simulink model "top_level_algo"  (R2022b)
settings: Solver=FixedStepAuto  StartTime=0.0  StopTime=inf  FixedStep=1e-3  RelTol=1e-3
values from neighbouring files (symbols this model uses):
  clk_period = 8    [Cals.m]
  gear_ratio = 10    [Cals.m]
  update_rate = 0.5    [Cals.m]
  Vdd = 3    [Cals.m]
undefined symbols (not defined in the file or in its folder): sigbuilder_block
libraries: simulink x24, stm32f4xxblockslib x12, embmathops x9, arduinolib x8, dspstat3 x4, dspswit3 x2
(part 2 of 3)

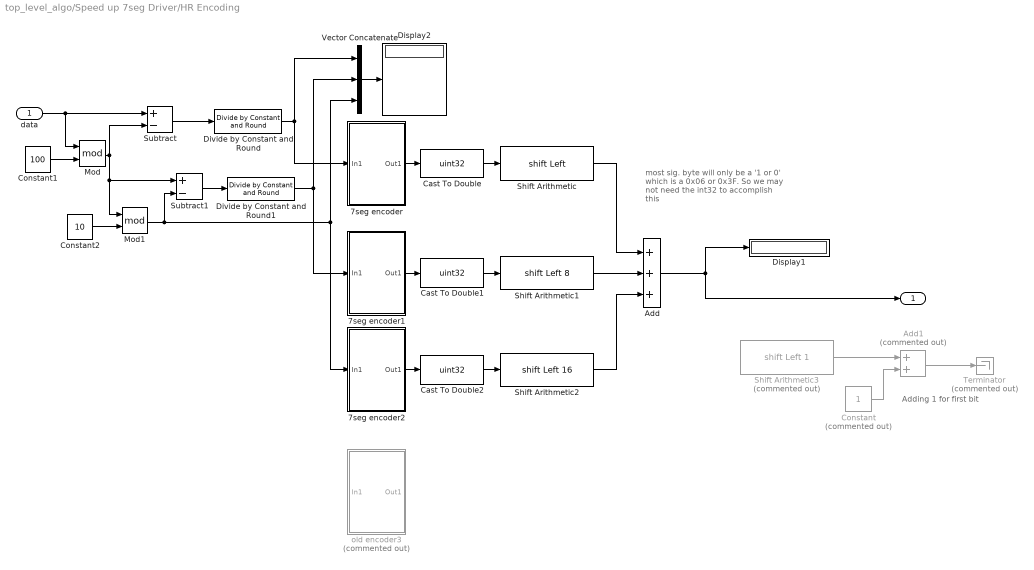
== system top_level_algo/Speed up 7seg Driver/HR Encoding ==
  note: Adding 1 for first bit
  note: most sig. byte will only be a '1 or 0' which is a 0x06 or 0x3F. So we may not need the int32 to accomplish this
  data : Inport
  7seg encoder : Subsystem
  7seg encoder1 : Subsystem
  7seg encoder2 : Subsystem
  Add : Sum  Inputs=+++
  Add1 : Sum  Commented=on
  Cast To Double : DataTypeConversion  OutDataTypeStr=uint32  SaturateOnIntegerOverflow=off  RndMeth=Floor
  Cast To Double1 : DataTypeConversion  OutDataTypeStr=uint32  SaturateOnIntegerOverflow=off  RndMeth=Floor
  Cast To Double2 : DataTypeConversion  OutDataTypeStr=uint32  SaturateOnIntegerOverflow=off  RndMeth=Floor
  Constant : Constant  Commented=on  OutDataTypeStr=uint32
  Constant1 : Constant  Value=100
  Constant2 : Constant  Value=10
  Display1 : Display
      settings: Format=hex (Stored Integer)
  Display2 : Display
  Divide by Constant and Round : embmathops/Divide by Constant and Round  Denominator=100  RoundingMethod=Floor  SimulateUsing=Code generation
  Divide by Constant and Round1 : embmathops/Divide by Constant and Round  Denominator=10  RoundingMethod=Floor  SimulateUsing=Code generation
  Mod : Math  Operator=mod
  Mod1 : Math  Operator=mod
  Shift Arithmetic : ArithShift  BitShiftDirection=Left
  Shift Arithmetic1 : ArithShift  BitShiftNumber=8  BitShiftDirection=Left
  Shift Arithmetic2 : ArithShift  BitShiftNumber=16  BitShiftDirection=Left
  Shift Arithmetic3 : ArithShift  Commented=on  BitShiftNumber=1  BitShiftDirection=Left
  Subtract : Sum  Inputs=+-
  Subtract1 : Sum  Inputs=+-
  Terminator : Terminator  Commented=on
  Vector Concatenate : Concatenate  NumInputs=3
  old encoder3 : Subsystem  Commented=on
  " " : Outport
  wires:
  Shift Arithmetic1/1 -> Add/2
  Mod1/1 -> Subtract1/2, Vector Concatenate/3, 7seg encoder2/1(In1)
  Mod/1 -> Subtract/2, Subtract1/1, Mod1/1
  7seg encoder/1(Out1) -> Cast To Double/1
  Subtract/1 -> Divide by Constant and Round/1
  Constant1/1 -> Mod/2
  Divide by Constant and Round/1 -> 7seg encoder/1(In1), Vector Concatenate/1
  Subtract1/1 -> Divide by Constant and Round1/1
  Cast To Double1/1 -> Shift Arithmetic1/1
  data/1 -> Mod/1, Subtract/1
  Add/1 -> Display1/1, " "/1
  Cast To Double/1 -> Shift Arithmetic/1
  Constant2/1 -> Mod1/2
  Vector Concatenate/1 -> Display2/1
  7seg encoder1/1(Out1) -> Cast To Double1/1
  Shift Arithmetic/1 -> Add/1
  Divide by Constant and Round1/1 -> Vector Concatenate/2, 7seg encoder1/1(In1)
  Shift Arithmetic2/1 -> Add/3
  7seg encoder2/1(Out1) -> Cast To Double2/1
  Cast To Double2/1 -> Shift Arithmetic2/1
  Constant/1 -> Add1/2
  Shift Arithmetic3/1 -> Add1/1
  Add1/1 -> Terminator/1

== system top_level_algo/Speed up 7seg Driver/clk ==
  In1 : Inport
  Cast To Single : DataTypeConversion  OutDataTypeStr=single  SaturateOnIntegerOverflow=off  RndMeth=Floor
  Compare To Constant : simulink/Logic and Bit Operations/Compare To Constant  relop=>=  const=1  OutDataTypeStr=boolean
  Constant : Constant
  Constant1 : Constant  Value=0
  Sum : Sum  Inputs=+-  InputSameDT=on  SaturateOnIntegerOverflow=on  OutDataTypeStr=Inherit: Same as first input
  Switch : Switch  Criteria=u2 > Threshold  SaturateOnIntegerOverflow=off  InputSameDT=off
  Unit Delay : UnitDelay  SampleTime=clk_period/2*1e-3  HasFrameUpgradeWarning=on
  Out1 : Outport
  wires:
  Sum/1 -> Switch/1, Out1/1
  Unit Delay/1 -> Sum/2
  In1/1 -> Cast To Single/1
  Cast To Single/1 -> Compare To Constant/1
  Constant1/1 -> Switch/3
  Compare To Constant/1 -> Switch/2
  Constant/1 -> Sum/1
  Switch/1 -> Unit Delay/1

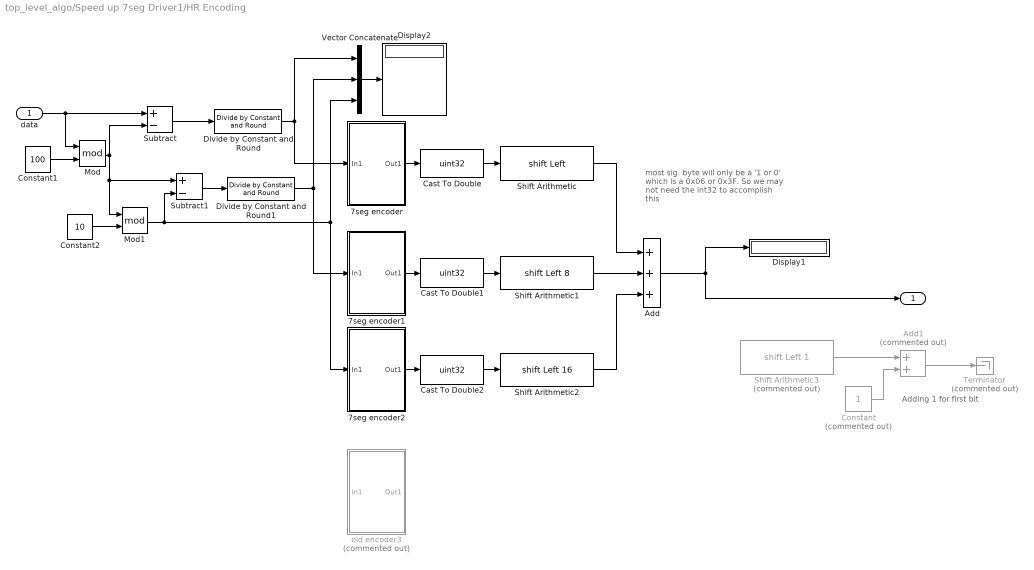
== system top_level_algo/Speed up 7seg Driver1/HR Encoding ==
  note: most sig. byte will only be a '1 or 0' which is a 0x06 or 0x3F. So we may not need the int32 to accomplish this
  note: Adding 1 for first bit
  data : Inport
  7seg encoder : Subsystem
  7seg encoder1 : Subsystem
  7seg encoder2 : Subsystem
  Add : Sum  Inputs=+++
  Add1 : Sum  Commented=on
  Cast To Double : DataTypeConversion  OutDataTypeStr=uint32  SaturateOnIntegerOverflow=off  RndMeth=Floor
  Cast To Double1 : DataTypeConversion  OutDataTypeStr=uint32  SaturateOnIntegerOverflow=off  RndMeth=Floor
  Cast To Double2 : DataTypeConversion  OutDataTypeStr=uint32  SaturateOnIntegerOverflow=off  RndMeth=Floor
  Constant : Constant  Commented=on  OutDataTypeStr=uint32
  Constant1 : Constant  Value=100
  Constant2 : Constant  Value=10
  Display1 : Display
      settings: Format=hex (Stored Integer)
  Display2 : Display
  Divide by Constant and Round : embmathops/Divide by Constant and Round  Denominator=100  RoundingMethod=Floor  SimulateUsing=Code generation
  Divide by Constant and Round1 : embmathops/Divide by Constant and Round  Denominator=10  RoundingMethod=Floor  SimulateUsing=Code generation
  Mod : Math  Operator=mod
  Mod1 : Math  Operator=mod
  Shift Arithmetic : ArithShift  BitShiftDirection=Left
  Shift Arithmetic1 : ArithShift  BitShiftNumber=8  BitShiftDirection=Left
  Shift Arithmetic2 : ArithShift  BitShiftNumber=16  BitShiftDirection=Left
  Shift Arithmetic3 : ArithShift  Commented=on  BitShiftNumber=1  BitShiftDirection=Left
  Subtract : Sum  Inputs=+-
  Subtract1 : Sum  Inputs=+-
  Terminator : Terminator  Commented=on
  Vector Concatenate : Concatenate  NumInputs=3
  old encoder3 : Subsystem  Commented=on
  " " : Outport
  wires:
  Add1/1 -> Terminator/1
  Shift Arithmetic3/1 -> Add1/1
  Constant/1 -> Add1/2
  Cast To Double2/1 -> Shift Arithmetic2/1
  7seg encoder2/1(Out1) -> Cast To Double2/1
  Shift Arithmetic2/1 -> Add/3
  Divide by Constant and Round1/1 -> 7seg encoder1/1(In1), Vector Concatenate/2
  Shift Arithmetic/1 -> Add/1
  7seg encoder1/1(Out1) -> Cast To Double1/1
  Vector Concatenate/1 -> Display2/1
  Constant2/1 -> Mod1/2
  Cast To Double/1 -> Shift Arithmetic/1
  Add/1 -> " "/1, Display1/1
  data/1 -> Subtract/1, Mod/1
  Cast To Double1/1 -> Shift Arithmetic1/1
  Subtract1/1 -> Divide by Constant and Round1/1
  Divide by Constant and Round/1 -> Vector Concatenate/1, 7seg encoder/1(In1)
  Constant1/1 -> Mod/2
  Subtract/1 -> Divide by Constant and Round/1
  7seg encoder/1(Out1) -> Cast To Double/1
  Mod/1 -> Mod1/1, Subtract1/1, Subtract/2
  Mod1/1 -> 7seg encoder2/1(In1), Vector Concatenate/3, Subtract1/2
  Shift Arithmetic1/1 -> Add/2

== system top_level_algo/Speed up 7seg Driver1/clk ==
  In1 : Inport
  Cast To Single : DataTypeConversion  OutDataTypeStr=single  SaturateOnIntegerOverflow=off  RndMeth=Floor
  Compare To Constant : simulink/Logic and Bit Operations/Compare To Constant  relop=>=  const=1  OutDataTypeStr=boolean
  Constant : Constant
  Constant1 : Constant  Value=0
  Sum : Sum  Inputs=+-  InputSameDT=on  SaturateOnIntegerOverflow=on  OutDataTypeStr=Inherit: Same as first input
  Switch : Switch  Criteria=u2 > Threshold  SaturateOnIntegerOverflow=off  InputSameDT=off
  Unit Delay : UnitDelay  SampleTime=clk_period/2*1e-3  HasFrameUpgradeWarning=on
  Out1 : Outport
  wires:
  Switch/1 -> Unit Delay/1
  Constant/1 -> Sum/1
  Compare To Constant/1 -> Switch/2
  Constant1/1 -> Switch/3
  Cast To Single/1 -> Compare To Constant/1
  In1/1 -> Cast To Single/1
  Unit Delay/1 -> Sum/2
  Sum/1 -> Out1/1, Switch/1

== system top_level_algo/7seg Driver/HR Encoding/7seg encoder ==
  In1 : Inport
  If Action Subsystem : Subsystem  TreatAsAtomicUnit=on
  If Action Subsystem1 : Subsystem  TreatAsAtomicUnit=on
  If Action Subsystem10 : Subsystem  TreatAsAtomicUnit=on
  If Action Subsystem2 : Subsystem  TreatAsAtomicUnit=on
  If Action Subsystem3 : Subsystem  TreatAsAtomicUnit=on
  If Action Subsystem4 : Subsystem  TreatAsAtomicUnit=on
  If Action Subsystem5 : Subsystem  TreatAsAtomicUnit=on
  If Action Subsystem6 : Subsystem  TreatAsAtomicUnit=on
  If Action Subsystem7 : Subsystem  TreatAsAtomicUnit=on
  If Action Subsystem8 : Subsystem  TreatAsAtomicUnit=on
  Merge : Merge  Inputs=10
  Switch Case : SwitchCase  CaseConditions={0,1,2,3,4,5,6,7,8,9}  ShowDefaultCase=off
  Out1 : Outport
  wires:
  If Action Subsystem3/1(Out1) -> Merge/4
  Switch Case/2 -> If Action Subsystem1/Action
  Switch Case/5 -> If Action Subsystem4/Action
  Switch Case/9 -> If Action Subsystem8/Action
  If Action Subsystem7/1(Out1) -> Merge/8
  Switch Case/6 -> If Action Subsystem5/Action
  If Action Subsystem4/1(Out1) -> Merge/5
  Switch Case/4 -> If Action Subsystem3/Action
  Switch Case/3 -> If Action Subsystem2/Action
  Switch Case/10 -> If Action Subsystem10/Action
  Switch Case/8 -> If Action Subsystem7/Action
  Switch Case/7 -> If Action Subsystem6/Action
  Switch Case/1 -> If Action Subsystem/Action
  If Action Subsystem6/1(Out1) -> Merge/7
  If Action Subsystem8/1(Out1) -> Merge/9
  If Action Subsystem5/1(Out1) -> Merge/6
  If Action Subsystem2/1(Out1) -> Merge/3
  If Action Subsystem10/1(Out1) -> Merge/10
  If Action Subsystem/1(Out1) -> Merge/1
  If Action Subsystem1/1(Out1) -> Merge/2
  In1/1 -> Switch Case/1
  Merge/1 -> Out1/1

== system top_level_algo/7seg Driver/HR Encoding/7seg encoder1 ==
  In1 : Inport
  If Action Subsystem : Subsystem  TreatAsAtomicUnit=on
  If Action Subsystem1 : Subsystem  TreatAsAtomicUnit=on
  If Action Subsystem10 : Subsystem  TreatAsAtomicUnit=on
  If Action Subsystem2 : Subsystem  TreatAsAtomicUnit=on
  If Action Subsystem3 : Subsystem  TreatAsAtomicUnit=on
  If Action Subsystem4 : Subsystem  TreatAsAtomicUnit=on
  If Action Subsystem5 : Subsystem  TreatAsAtomicUnit=on
  If Action Subsystem6 : Subsystem  TreatAsAtomicUnit=on
  If Action Subsystem7 : Subsystem  TreatAsAtomicUnit=on
  If Action Subsystem8 : Subsystem  TreatAsAtomicUnit=on
  Merge : Merge  Inputs=10
  Switch Case : SwitchCase  CaseConditions={0,1,2,3,4,5,6,7,8,9}  ShowDefaultCase=off
  Out1 : Outport
  wires:
  If Action Subsystem3/1(Out1) -> Merge/4
  Switch Case/2 -> If Action Subsystem1/Action
  Switch Case/5 -> If Action Subsystem4/Action
  Switch Case/9 -> If Action Subsystem8/Action
  If Action Subsystem7/1(Out1) -> Merge/8
  Switch Case/6 -> If Action Subsystem5/Action
  If Action Subsystem4/1(Out1) -> Merge/5
  Switch Case/4 -> If Action Subsystem3/Action
  Switch Case/3 -> If Action Subsystem2/Action
  Switch Case/10 -> If Action Subsystem10/Action
  Switch Case/8 -> If Action Subsystem7/Action
  Switch Case/7 -> If Action Subsystem6/Action
  Switch Case/1 -> If Action Subsystem/Action
  If Action Subsystem6/1(Out1) -> Merge/7
  If Action Subsystem8/1(Out1) -> Merge/9
  If Action Subsystem5/1(Out1) -> Merge/6
  If Action Subsystem2/1(Out1) -> Merge/3
  If Action Subsystem10/1(Out1) -> Merge/10
  If Action Subsystem/1(Out1) -> Merge/1
  If Action Subsystem1/1(Out1) -> Merge/2
  In1/1 -> Switch Case/1
  Merge/1 -> Out1/1

== system top_level_algo/7seg Driver/HR Encoding/7seg encoder2 ==
  In1 : Inport
  If Action Subsystem : Subsystem  TreatAsAtomicUnit=on
  If Action Subsystem1 : Subsystem  TreatAsAtomicUnit=on
  If Action Subsystem10 : Subsystem  TreatAsAtomicUnit=on
  If Action Subsystem2 : Subsystem  TreatAsAtomicUnit=on
  If Action Subsystem3 : Subsystem  TreatAsAtomicUnit=on
  If Action Subsystem4 : Subsystem  TreatAsAtomicUnit=on
  If Action Subsystem5 : Subsystem  TreatAsAtomicUnit=on
  If Action Subsystem6 : Subsystem  TreatAsAtomicUnit=on
  If Action Subsystem7 : Subsystem  TreatAsAtomicUnit=on
  If Action Subsystem8 : Subsystem  TreatAsAtomicUnit=on
  Merge : Merge  Inputs=10
  Switch Case : SwitchCase  CaseConditions={0,1,2,3,4,5,6,7,8,9}  ShowDefaultCase=off
  Out1 : Outport
  wires:
  If Action Subsystem3/1(Out1) -> Merge/4
  Switch Case/2 -> If Action Subsystem1/Action
  Switch Case/5 -> If Action Subsystem4/Action
  Switch Case/9 -> If Action Subsystem8/Action
  If Action Subsystem7/1(Out1) -> Merge/8
  Switch Case/6 -> If Action Subsystem5/Action
  If Action Subsystem4/1(Out1) -> Merge/5
  Switch Case/4 -> If Action Subsystem3/Action
  Switch Case/3 -> If Action Subsystem2/Action
  Switch Case/10 -> If Action Subsystem10/Action
  Switch Case/8 -> If Action Subsystem7/Action
  Switch Case/7 -> If Action Subsystem6/Action
  Switch Case/1 -> If Action Subsystem/Action
  If Action Subsystem6/1(Out1) -> Merge/7
  If Action Subsystem8/1(Out1) -> Merge/9
  If Action Subsystem5/1(Out1) -> Merge/6
  If Action Subsystem2/1(Out1) -> Merge/3
  If Action Subsystem10/1(Out1) -> Merge/10
  If Action Subsystem/1(Out1) -> Merge/1
  If Action Subsystem1/1(Out1) -> Merge/2
  In1/1 -> Switch Case/1
  Merge/1 -> Out1/1

== system top_level_algo/7seg Driver/HR Encoding/old encoder3 ==
  In1 : Inport
  If Action Subsystem : Subsystem  TreatAsAtomicUnit=on
  If Action Subsystem1 : Subsystem  TreatAsAtomicUnit=on
  If Action Subsystem10 : Subsystem  TreatAsAtomicUnit=on
  If Action Subsystem2 : Subsystem  TreatAsAtomicUnit=on
  If Action Subsystem3 : Subsystem  TreatAsAtomicUnit=on
  If Action Subsystem4 : Subsystem  TreatAsAtomicUnit=on
  If Action Subsystem5 : Subsystem  TreatAsAtomicUnit=on
  If Action Subsystem6 : Subsystem  TreatAsAtomicUnit=on
  If Action Subsystem7 : Subsystem  TreatAsAtomicUnit=on
  If Action Subsystem8 : Subsystem  TreatAsAtomicUnit=on
  Merge : Merge  Inputs=10
  Switch Case : SwitchCase  CaseConditions={0,1,2,3,4,5,6,7,8,9}  ShowDefaultCase=off
  Out1 : Outport
  wires:
  If Action Subsystem3/1(Out1) -> Merge/4
  Switch Case/2 -> If Action Subsystem1/Action
  Switch Case/5 -> If Action Subsystem4/Action
  Switch Case/9 -> If Action Subsystem8/Action
  If Action Subsystem7/1(Out1) -> Merge/8
  Switch Case/6 -> If Action Subsystem5/Action
  If Action Subsystem4/1(Out1) -> Merge/5
  Switch Case/4 -> If Action Subsystem3/Action
  Switch Case/3 -> If Action Subsystem2/Action
  Switch Case/10 -> If Action Subsystem10/Action
  Switch Case/8 -> If Action Subsystem7/Action
  Switch Case/7 -> If Action Subsystem6/Action
  Switch Case/1 -> If Action Subsystem/Action
  If Action Subsystem6/1(Out1) -> Merge/7
  If Action Subsystem8/1(Out1) -> Merge/9
  If Action Subsystem5/1(Out1) -> Merge/6
  If Action Subsystem2/1(Out1) -> Merge/3
  If Action Subsystem10/1(Out1) -> Merge/10
  If Action Subsystem/1(Out1) -> Merge/1
  If Action Subsystem1/1(Out1) -> Merge/2
  In1/1 -> Switch Case/1
  Merge/1 -> Out1/1

== system top_level_algo/7seg Driver2/HR Encoding/7seg encoder ==
  In1 : Inport
  If Action Subsystem : Subsystem  TreatAsAtomicUnit=on
  If Action Subsystem1 : Subsystem  TreatAsAtomicUnit=on
  If Action Subsystem10 : Subsystem  TreatAsAtomicUnit=on
  If Action Subsystem2 : Subsystem  TreatAsAtomicUnit=on
  If Action Subsystem3 : Subsystem  TreatAsAtomicUnit=on
  If Action Subsystem4 : Subsystem  TreatAsAtomicUnit=on
  If Action Subsystem5 : Subsystem  TreatAsAtomicUnit=on
  If Action Subsystem6 : Subsystem  TreatAsAtomicUnit=on
  If Action Subsystem7 : Subsystem  TreatAsAtomicUnit=on
  If Action Subsystem8 : Subsystem  TreatAsAtomicUnit=on
  Merge : Merge  Inputs=10
  Switch Case : SwitchCase  CaseConditions={0,1,2,3,4,5,6,7,8,9}  ShowDefaultCase=off
  Out1 : Outport
  wires:
  If Action Subsystem3/1(Out1) -> Merge/4
  Switch Case/2 -> If Action Subsystem1/Action
  Switch Case/5 -> If Action Subsystem4/Action
  Switch Case/9 -> If Action Subsystem8/Action
  If Action Subsystem7/1(Out1) -> Merge/8
  Switch Case/6 -> If Action Subsystem5/Action
  If Action Subsystem4/1(Out1) -> Merge/5
  Switch Case/4 -> If Action Subsystem3/Action
  Switch Case/3 -> If Action Subsystem2/Action
  Switch Case/10 -> If Action Subsystem10/Action
  Switch Case/8 -> If Action Subsystem7/Action
  Switch Case/7 -> If Action Subsystem6/Action
  Switch Case/1 -> If Action Subsystem/Action
  If Action Subsystem6/1(Out1) -> Merge/7
  If Action Subsystem8/1(Out1) -> Merge/9
  If Action Subsystem5/1(Out1) -> Merge/6
  If Action Subsystem2/1(Out1) -> Merge/3
  If Action Subsystem10/1(Out1) -> Merge/10
  If Action Subsystem/1(Out1) -> Merge/1
  If Action Subsystem1/1(Out1) -> Merge/2
  In1/1 -> Switch Case/1
  Merge/1 -> Out1/1

== system top_level_algo/7seg Driver2/HR Encoding/7seg encoder1 ==
  In1 : Inport
  If Action Subsystem : Subsystem  TreatAsAtomicUnit=on
  If Action Subsystem1 : Subsystem  TreatAsAtomicUnit=on
  If Action Subsystem10 : Subsystem  TreatAsAtomicUnit=on
  If Action Subsystem2 : Subsystem  TreatAsAtomicUnit=on
  If Action Subsystem3 : Subsystem  TreatAsAtomicUnit=on
  If Action Subsystem4 : Subsystem  TreatAsAtomicUnit=on
  If Action Subsystem5 : Subsystem  TreatAsAtomicUnit=on
  If Action Subsystem6 : Subsystem  TreatAsAtomicUnit=on
  If Action Subsystem7 : Subsystem  TreatAsAtomicUnit=on
  If Action Subsystem8 : Subsystem  TreatAsAtomicUnit=on
  Merge : Merge  Inputs=10
  Switch Case : SwitchCase  CaseConditions={0,1,2,3,4,5,6,7,8,9}  ShowDefaultCase=off
  Out1 : Outport
  wires:
  If Action Subsystem3/1(Out1) -> Merge/4
  Switch Case/2 -> If Action Subsystem1/Action
  Switch Case/5 -> If Action Subsystem4/Action
  Switch Case/9 -> If Action Subsystem8/Action
  If Action Subsystem7/1(Out1) -> Merge/8
  Switch Case/6 -> If Action Subsystem5/Action
  If Action Subsystem4/1(Out1) -> Merge/5
  Switch Case/4 -> If Action Subsystem3/Action
  Switch Case/3 -> If Action Subsystem2/Action
  Switch Case/10 -> If Action Subsystem10/Action
  Switch Case/8 -> If Action Subsystem7/Action
  Switch Case/7 -> If Action Subsystem6/Action
  Switch Case/1 -> If Action Subsystem/Action
  If Action Subsystem6/1(Out1) -> Merge/7
  If Action Subsystem8/1(Out1) -> Merge/9
  If Action Subsystem5/1(Out1) -> Merge/6
  If Action Subsystem2/1(Out1) -> Merge/3
  If Action Subsystem10/1(Out1) -> Merge/10
  If Action Subsystem/1(Out1) -> Merge/1
  If Action Subsystem1/1(Out1) -> Merge/2
  In1/1 -> Switch Case/1
  Merge/1 -> Out1/1

== system top_level_algo/7seg Driver2/HR Encoding/7seg encoder2 ==
  In1 : Inport
  If Action Subsystem : Subsystem  TreatAsAtomicUnit=on
  If Action Subsystem1 : Subsystem  TreatAsAtomicUnit=on
  If Action Subsystem10 : Subsystem  TreatAsAtomicUnit=on
  If Action Subsystem2 : Subsystem  TreatAsAtomicUnit=on
  If Action Subsystem3 : Subsystem  TreatAsAtomicUnit=on
  If Action Subsystem4 : Subsystem  TreatAsAtomicUnit=on
  If Action Subsystem5 : Subsystem  TreatAsAtomicUnit=on
  If Action Subsystem6 : Subsystem  TreatAsAtomicUnit=on
  If Action Subsystem7 : Subsystem  TreatAsAtomicUnit=on
  If Action Subsystem8 : Subsystem  TreatAsAtomicUnit=on
  Merge : Merge  Inputs=10
  Switch Case : SwitchCase  CaseConditions={0,1,2,3,4,5,6,7,8,9}  ShowDefaultCase=off
  Out1 : Outport
  wires:
  If Action Subsystem3/1(Out1) -> Merge/4
  Switch Case/2 -> If Action Subsystem1/Action
  Switch Case/5 -> If Action Subsystem4/Action
  Switch Case/9 -> If Action Subsystem8/Action
  If Action Subsystem7/1(Out1) -> Merge/8
  Switch Case/6 -> If Action Subsystem5/Action
  If Action Subsystem4/1(Out1) -> Merge/5
  Switch Case/4 -> If Action Subsystem3/Action
  Switch Case/3 -> If Action Subsystem2/Action
  Switch Case/10 -> If Action Subsystem10/Action
  Switch Case/8 -> If Action Subsystem7/Action
  Switch Case/7 -> If Action Subsystem6/Action
  Switch Case/1 -> If Action Subsystem/Action
  If Action Subsystem6/1(Out1) -> Merge/7
  If Action Subsystem8/1(Out1) -> Merge/9
  If Action Subsystem5/1(Out1) -> Merge/6
  If Action Subsystem2/1(Out1) -> Merge/3
  If Action Subsystem10/1(Out1) -> Merge/10
  If Action Subsystem/1(Out1) -> Merge/1
  If Action Subsystem1/1(Out1) -> Merge/2
  In1/1 -> Switch Case/1
  Merge/1 -> Out1/1

== system top_level_algo/7seg Driver2/HR Encoding/old encoder3 ==
  In1 : Inport
  If Action Subsystem : Subsystem  TreatAsAtomicUnit=on
  If Action Subsystem1 : Subsystem  TreatAsAtomicUnit=on
  If Action Subsystem10 : Subsystem  TreatAsAtomicUnit=on
  If Action Subsystem2 : Subsystem  TreatAsAtomicUnit=on
  If Action Subsystem3 : Subsystem  TreatAsAtomicUnit=on
  If Action Subsystem4 : Subsystem  TreatAsAtomicUnit=on
  If Action Subsystem5 : Subsystem  TreatAsAtomicUnit=on
  If Action Subsystem6 : Subsystem  TreatAsAtomicUnit=on
  If Action Subsystem7 : Subsystem  TreatAsAtomicUnit=on
  If Action Subsystem8 : Subsystem  TreatAsAtomicUnit=on
  Merge : Merge  Inputs=10
  Switch Case : SwitchCase  CaseConditions={0,1,2,3,4,5,6,7,8,9}  ShowDefaultCase=off
  Out1 : Outport
  wires:
  If Action Subsystem3/1(Out1) -> Merge/4
  Switch Case/2 -> If Action Subsystem1/Action
  Switch Case/5 -> If Action Subsystem4/Action
  Switch Case/9 -> If Action Subsystem8/Action
  If Action Subsystem7/1(Out1) -> Merge/8
  Switch Case/6 -> If Action Subsystem5/Action
  If Action Subsystem4/1(Out1) -> Merge/5
  Switch Case/4 -> If Action Subsystem3/Action
  Switch Case/3 -> If Action Subsystem2/Action
  Switch Case/10 -> If Action Subsystem10/Action
  Switch Case/8 -> If Action Subsystem7/Action
  Switch Case/7 -> If Action Subsystem6/Action
  Switch Case/1 -> If Action Subsystem/Action
  If Action Subsystem6/1(Out1) -> Merge/7
  If Action Subsystem8/1(Out1) -> Merge/9
  If Action Subsystem5/1(Out1) -> Merge/6
  If Action Subsystem2/1(Out1) -> Merge/3
  If Action Subsystem10/1(Out1) -> Merge/10
  If Action Subsystem/1(Out1) -> Merge/1
  If Action Subsystem1/1(Out1) -> Merge/2
  In1/1 -> Switch Case/1
  Merge/1 -> Out1/1

== system top_level_algo/Hardware Hiding/force min to zero/If Action Subsystem ==
  In1 : Inport
  Action Port : ActionPort  ActionPortLabel=if(u1 < 0)
  Out1 : Outport
  wires:
  In1/1 -> Out1/1

== system top_level_algo/Hardware Hiding/force min to zero/If Action Subsystem1 ==
  In1 : Inport
  Action Port : ActionPort  ActionPortLabel=else
  Out1 : Outport
  wires:
  In1/1 -> Out1/1

== system top_level_algo/MinMax/force min to zero/If Action Subsystem ==
  In1 : Inport
  Action Port : ActionPort  ActionPortLabel=if(u1 < 0)
  Out1 : Outport
  wires:
  In1/1 -> Out1/1

== system top_level_algo/MinMax/force min to zero/If Action Subsystem1 ==
  In1 : Inport
  Action Port : ActionPort  ActionPortLabel=else
  Out1 : Outport
  wires:
  In1/1 -> Out1/1

== system top_level_algo/Speed up 7seg Driver/HR Encoding/7seg encoder ==
  In1 : Inport
  If Action Subsystem : Subsystem  TreatAsAtomicUnit=on
  If Action Subsystem1 : Subsystem  TreatAsAtomicUnit=on
  If Action Subsystem10 : Subsystem  TreatAsAtomicUnit=on
  If Action Subsystem2 : Subsystem  TreatAsAtomicUnit=on
  If Action Subsystem3 : Subsystem  TreatAsAtomicUnit=on
  If Action Subsystem4 : Subsystem  TreatAsAtomicUnit=on
  If Action Subsystem5 : Subsystem  TreatAsAtomicUnit=on
  If Action Subsystem6 : Subsystem  TreatAsAtomicUnit=on
  If Action Subsystem7 : Subsystem  TreatAsAtomicUnit=on
  If Action Subsystem8 : Subsystem  TreatAsAtomicUnit=on
  Merge : Merge  Inputs=10
  Switch Case : SwitchCase  CaseConditions={0,1,2,3,4,5,6,7,8,9}  ShowDefaultCase=off
  Out1 : Outport
  wires:
  If Action Subsystem3/1(Out1) -> Merge/4
  Switch Case/2 -> If Action Subsystem1/Action
  Switch Case/5 -> If Action Subsystem4/Action
  Switch Case/9 -> If Action Subsystem8/Action
  If Action Subsystem7/1(Out1) -> Merge/8
  Switch Case/6 -> If Action Subsystem5/Action
  If Action Subsystem4/1(Out1) -> Merge/5
  Switch Case/4 -> If Action Subsystem3/Action
  Switch Case/3 -> If Action Subsystem2/Action
  Switch Case/10 -> If Action Subsystem10/Action
  Switch Case/8 -> If Action Subsystem7/Action
  Switch Case/7 -> If Action Subsystem6/Action
  Switch Case/1 -> If Action Subsystem/Action
  If Action Subsystem6/1(Out1) -> Merge/7
  If Action Subsystem8/1(Out1) -> Merge/9
  If Action Subsystem5/1(Out1) -> Merge/6
  If Action Subsystem2/1(Out1) -> Merge/3
  If Action Subsystem10/1(Out1) -> Merge/10
  If Action Subsystem/1(Out1) -> Merge/1
  If Action Subsystem1/1(Out1) -> Merge/2
  In1/1 -> Switch Case/1
  Merge/1 -> Out1/1

== system top_level_algo/Speed up 7seg Driver/HR Encoding/7seg encoder1 ==
  In1 : Inport
  If Action Subsystem : Subsystem  TreatAsAtomicUnit=on
  If Action Subsystem1 : Subsystem  TreatAsAtomicUnit=on
  If Action Subsystem10 : Subsystem  TreatAsAtomicUnit=on
  If Action Subsystem2 : Subsystem  TreatAsAtomicUnit=on
  If Action Subsystem3 : Subsystem  TreatAsAtomicUnit=on
  If Action Subsystem4 : Subsystem  TreatAsAtomicUnit=on
  If Action Subsystem5 : Subsystem  TreatAsAtomicUnit=on
  If Action Subsystem6 : Subsystem  TreatAsAtomicUnit=on
  If Action Subsystem7 : Subsystem  TreatAsAtomicUnit=on
  If Action Subsystem8 : Subsystem  TreatAsAtomicUnit=on
  Merge : Merge  Inputs=10
  Switch Case : SwitchCase  CaseConditions={0,1,2,3,4,5,6,7,8,9}  ShowDefaultCase=off
  Out1 : Outport
  wires:
  If Action Subsystem3/1(Out1) -> Merge/4
  Switch Case/2 -> If Action Subsystem1/Action
  Switch Case/5 -> If Action Subsystem4/Action
  Switch Case/9 -> If Action Subsystem8/Action
  If Action Subsystem7/1(Out1) -> Merge/8
  Switch Case/6 -> If Action Subsystem5/Action
  If Action Subsystem4/1(Out1) -> Merge/5
  Switch Case/4 -> If Action Subsystem3/Action
  Switch Case/3 -> If Action Subsystem2/Action
  Switch Case/10 -> If Action Subsystem10/Action
  Switch Case/8 -> If Action Subsystem7/Action
  Switch Case/7 -> If Action Subsystem6/Action
  Switch Case/1 -> If Action Subsystem/Action
  If Action Subsystem6/1(Out1) -> Merge/7
  If Action Subsystem8/1(Out1) -> Merge/9
  If Action Subsystem5/1(Out1) -> Merge/6
  If Action Subsystem2/1(Out1) -> Merge/3
  If Action Subsystem10/1(Out1) -> Merge/10
  If Action Subsystem/1(Out1) -> Merge/1
  If Action Subsystem1/1(Out1) -> Merge/2
  In1/1 -> Switch Case/1
  Merge/1 -> Out1/1

== system top_level_algo/Speed up 7seg Driver/HR Encoding/7seg encoder2 ==
  In1 : Inport
  If Action Subsystem : Subsystem  TreatAsAtomicUnit=on
  If Action Subsystem1 : Subsystem  TreatAsAtomicUnit=on
  If Action Subsystem10 : Subsystem  TreatAsAtomicUnit=on
  If Action Subsystem2 : Subsystem  TreatAsAtomicUnit=on
  If Action Subsystem3 : Subsystem  TreatAsAtomicUnit=on
  If Action Subsystem4 : Subsystem  TreatAsAtomicUnit=on
  If Action Subsystem5 : Subsystem  TreatAsAtomicUnit=on
  If Action Subsystem6 : Subsystem  TreatAsAtomicUnit=on
  If Action Subsystem7 : Subsystem  TreatAsAtomicUnit=on
  If Action Subsystem8 : Subsystem  TreatAsAtomicUnit=on
  Merge : Merge  Inputs=10
  Switch Case : SwitchCase  CaseConditions={0,1,2,3,4,5,6,7,8,9}  ShowDefaultCase=off
  Out1 : Outport
  wires:
  If Action Subsystem3/1(Out1) -> Merge/4
  Switch Case/2 -> If Action Subsystem1/Action
  Switch Case/5 -> If Action Subsystem4/Action
  Switch Case/9 -> If Action Subsystem8/Action
  If Action Subsystem7/1(Out1) -> Merge/8
  Switch Case/6 -> If Action Subsystem5/Action
  If Action Subsystem4/1(Out1) -> Merge/5
  Switch Case/4 -> If Action Subsystem3/Action
  Switch Case/3 -> If Action Subsystem2/Action
  Switch Case/10 -> If Action Subsystem10/Action
  Switch Case/8 -> If Action Subsystem7/Action
  Switch Case/7 -> If Action Subsystem6/Action
  Switch Case/1 -> If Action Subsystem/Action
  If Action Subsystem6/1(Out1) -> Merge/7
  If Action Subsystem8/1(Out1) -> Merge/9
  If Action Subsystem5/1(Out1) -> Merge/6
  If Action Subsystem2/1(Out1) -> Merge/3
  If Action Subsystem10/1(Out1) -> Merge/10
  If Action Subsystem/1(Out1) -> Merge/1
  If Action Subsystem1/1(Out1) -> Merge/2
  In1/1 -> Switch Case/1
  Merge/1 -> Out1/1

== system top_level_algo/Speed up 7seg Driver/HR Encoding/old encoder3 ==
  In1 : Inport
  If Action Subsystem : Subsystem  TreatAsAtomicUnit=on
  If Action Subsystem1 : Subsystem  TreatAsAtomicUnit=on
  If Action Subsystem10 : Subsystem  TreatAsAtomicUnit=on
  If Action Subsystem2 : Subsystem  TreatAsAtomicUnit=on
  If Action Subsystem3 : Subsystem  TreatAsAtomicUnit=on
  If Action Subsystem4 : Subsystem  TreatAsAtomicUnit=on
  If Action Subsystem5 : Subsystem  TreatAsAtomicUnit=on
  If Action Subsystem6 : Subsystem  TreatAsAtomicUnit=on
  If Action Subsystem7 : Subsystem  TreatAsAtomicUnit=on
  If Action Subsystem8 : Subsystem  TreatAsAtomicUnit=on
  Merge : Merge  Inputs=10
  Switch Case : SwitchCase  CaseConditions={0,1,2,3,4,5,6,7,8,9}  ShowDefaultCase=off
  Out1 : Outport
  wires:
  If Action Subsystem3/1(Out1) -> Merge/4
  Switch Case/2 -> If Action Subsystem1/Action
  Switch Case/5 -> If Action Subsystem4/Action
  Switch Case/9 -> If Action Subsystem8/Action
  If Action Subsystem7/1(Out1) -> Merge/8
  Switch Case/6 -> If Action Subsystem5/Action
  If Action Subsystem4/1(Out1) -> Merge/5
  Switch Case/4 -> If Action Subsystem3/Action
  Switch Case/3 -> If Action Subsystem2/Action
  Switch Case/10 -> If Action Subsystem10/Action
  Switch Case/8 -> If Action Subsystem7/Action
  Switch Case/7 -> If Action Subsystem6/Action
  Switch Case/1 -> If Action Subsystem/Action
  If Action Subsystem6/1(Out1) -> Merge/7
  If Action Subsystem8/1(Out1) -> Merge/9
  If Action Subsystem5/1(Out1) -> Merge/6
  If Action Subsystem2/1(Out1) -> Merge/3
  If Action Subsystem10/1(Out1) -> Merge/10
  If Action Subsystem/1(Out1) -> Merge/1
  If Action Subsystem1/1(Out1) -> Merge/2
  In1/1 -> Switch Case/1
  Merge/1 -> Out1/1

== system top_level_algo/Speed up 7seg Driver1/HR Encoding/7seg encoder ==
  In1 : Inport
  If Action Subsystem : Subsystem  TreatAsAtomicUnit=on
  If Action Subsystem1 : Subsystem  TreatAsAtomicUnit=on
  If Action Subsystem10 : Subsystem  TreatAsAtomicUnit=on
  If Action Subsystem2 : Subsystem  TreatAsAtomicUnit=on
  If Action Subsystem3 : Subsystem  TreatAsAtomicUnit=on
  If Action Subsystem4 : Subsystem  TreatAsAtomicUnit=on
  If Action Subsystem5 : Subsystem  TreatAsAtomicUnit=on
  If Action Subsystem6 : Subsystem  TreatAsAtomicUnit=on
  If Action Subsystem7 : Subsystem  TreatAsAtomicUnit=on
  If Action Subsystem8 : Subsystem  TreatAsAtomicUnit=on
  Merge : Merge  Inputs=10
  Switch Case : SwitchCase  CaseConditions={0,1,2,3,4,5,6,7,8,9}  ShowDefaultCase=off
  Out1 : Outport
  wires:
  Merge/1 -> Out1/1
  In1/1 -> Switch Case/1
  If Action Subsystem1/1(Out1) -> Merge/2
  If Action Subsystem/1(Out1) -> Merge/1
  If Action Subsystem10/1(Out1) -> Merge/10
  If Action Subsystem2/1(Out1) -> Merge/3
  If Action Subsystem5/1(Out1) -> Merge/6
  If Action Subsystem8/1(Out1) -> Merge/9
  If Action Subsystem6/1(Out1) -> Merge/7
  Switch Case/1 -> If Action Subsystem/Action
  Switch Case/7 -> If Action Subsystem6/Action
  Switch Case/8 -> If Action Subsystem7/Action
  Switch Case/10 -> If Action Subsystem10/Action
  Switch Case/3 -> If Action Subsystem2/Action
  Switch Case/4 -> If Action Subsystem3/Action
  If Action Subsystem4/1(Out1) -> Merge/5
  Switch Case/6 -> If Action Subsystem5/Action
  If Action Subsystem7/1(Out1) -> Merge/8
  Switch Case/9 -> If Action Subsystem8/Action
  Switch Case/5 -> If Action Subsystem4/Action
  Switch Case/2 -> If Action Subsystem1/Action
  If Action Subsystem3/1(Out1) -> Merge/4

== system top_level_algo/Speed up 7seg Driver1/HR Encoding/7seg encoder1 ==
  In1 : Inport
  If Action Subsystem : Subsystem  TreatAsAtomicUnit=on
  If Action Subsystem1 : Subsystem  TreatAsAtomicUnit=on
  If Action Subsystem10 : Subsystem  TreatAsAtomicUnit=on
  If Action Subsystem2 : Subsystem  TreatAsAtomicUnit=on
  If Action Subsystem3 : Subsystem  TreatAsAtomicUnit=on
  If Action Subsystem4 : Subsystem  TreatAsAtomicUnit=on
  If Action Subsystem5 : Subsystem  TreatAsAtomicUnit=on
  If Action Subsystem6 : Subsystem  TreatAsAtomicUnit=on
  If Action Subsystem7 : Subsystem  TreatAsAtomicUnit=on
  If Action Subsystem8 : Subsystem  TreatAsAtomicUnit=on
  Merge : Merge  Inputs=10
  Switch Case : SwitchCase  CaseConditions={0,1,2,3,4,5,6,7,8,9}  ShowDefaultCase=off
  Out1 : Outport
  wires:
  Merge/1 -> Out1/1
  In1/1 -> Switch Case/1
  If Action Subsystem1/1(Out1) -> Merge/2
  If Action Subsystem/1(Out1) -> Merge/1
  If Action Subsystem10/1(Out1) -> Merge/10
  If Action Subsystem2/1(Out1) -> Merge/3
  If Action Subsystem5/1(Out1) -> Merge/6
  If Action Subsystem8/1(Out1) -> Merge/9
  If Action Subsystem6/1(Out1) -> Merge/7
  Switch Case/1 -> If Action Subsystem/Action
  Switch Case/7 -> If Action Subsystem6/Action
  Switch Case/8 -> If Action Subsystem7/Action
  Switch Case/10 -> If Action Subsystem10/Action
  Switch Case/3 -> If Action Subsystem2/Action
  Switch Case/4 -> If Action Subsystem3/Action
  If Action Subsystem4/1(Out1) -> Merge/5
  Switch Case/6 -> If Action Subsystem5/Action
  If Action Subsystem7/1(Out1) -> Merge/8
  Switch Case/9 -> If Action Subsystem8/Action
  Switch Case/5 -> If Action Subsystem4/Action
  Switch Case/2 -> If Action Subsystem1/Action
  If Action Subsystem3/1(Out1) -> Merge/4

== system top_level_algo/Speed up 7seg Driver1/HR Encoding/7seg encoder2 ==
  In1 : Inport
  If Action Subsystem : Subsystem  TreatAsAtomicUnit=on
  If Action Subsystem1 : Subsystem  TreatAsAtomicUnit=on
  If Action Subsystem10 : Subsystem  TreatAsAtomicUnit=on
  If Action Subsystem2 : Subsystem  TreatAsAtomicUnit=on
  If Action Subsystem3 : Subsystem  TreatAsAtomicUnit=on
  If Action Subsystem4 : Subsystem  TreatAsAtomicUnit=on
  If Action Subsystem5 : Subsystem  TreatAsAtomicUnit=on
  If Action Subsystem6 : Subsystem  TreatAsAtomicUnit=on
  If Action Subsystem7 : Subsystem  TreatAsAtomicUnit=on
  If Action Subsystem8 : Subsystem  TreatAsAtomicUnit=on
  Merge : Merge  Inputs=10
  Switch Case : SwitchCase  CaseConditions={0,1,2,3,4,5,6,7,8,9}  ShowDefaultCase=off
  Out1 : Outport
  wires:
  Merge/1 -> Out1/1
  In1/1 -> Switch Case/1
  If Action Subsystem1/1(Out1) -> Merge/2
  If Action Subsystem/1(Out1) -> Merge/1
  If Action Subsystem10/1(Out1) -> Merge/10
  If Action Subsystem2/1(Out1) -> Merge/3
  If Action Subsystem5/1(Out1) -> Merge/6
  If Action Subsystem8/1(Out1) -> Merge/9
  If Action Subsystem6/1(Out1) -> Merge/7
  Switch Case/1 -> If Action Subsystem/Action
  Switch Case/7 -> If Action Subsystem6/Action
  Switch Case/8 -> If Action Subsystem7/Action
  Switch Case/10 -> If Action Subsystem10/Action
  Switch Case/3 -> If Action Subsystem2/Action
  Switch Case/4 -> If Action Subsystem3/Action
  If Action Subsystem4/1(Out1) -> Merge/5
  Switch Case/6 -> If Action Subsystem5/Action
  If Action Subsystem7/1(Out1) -> Merge/8
  Switch Case/9 -> If Action Subsystem8/Action
  Switch Case/5 -> If Action Subsystem4/Action
  Switch Case/2 -> If Action Subsystem1/Action
  If Action Subsystem3/1(Out1) -> Merge/4

== system top_level_algo/Speed up 7seg Driver1/HR Encoding/old encoder3 ==
  In1 : Inport
  If Action Subsystem : Subsystem  TreatAsAtomicUnit=on
  If Action Subsystem1 : Subsystem  TreatAsAtomicUnit=on
  If Action Subsystem10 : Subsystem  TreatAsAtomicUnit=on
  If Action Subsystem2 : Subsystem  TreatAsAtomicUnit=on
  If Action Subsystem3 : Subsystem  TreatAsAtomicUnit=on
  If Action Subsystem4 : Subsystem  TreatAsAtomicUnit=on
  If Action Subsystem5 : Subsystem  TreatAsAtomicUnit=on
  If Action Subsystem6 : Subsystem  TreatAsAtomicUnit=on
  If Action Subsystem7 : Subsystem  TreatAsAtomicUnit=on
  If Action Subsystem8 : Subsystem  TreatAsAtomicUnit=on
  Merge : Merge  Inputs=10
  Switch Case : SwitchCase  CaseConditions={0,1,2,3,4,5,6,7,8,9}  ShowDefaultCase=off
  Out1 : Outport
  wires:
  Merge/1 -> Out1/1
  In1/1 -> Switch Case/1
  If Action Subsystem1/1(Out1) -> Merge/2
  If Action Subsystem/1(Out1) -> Merge/1
  If Action Subsystem10/1(Out1) -> Merge/10
  If Action Subsystem2/1(Out1) -> Merge/3
  If Action Subsystem5/1(Out1) -> Merge/6
  If Action Subsystem8/1(Out1) -> Merge/9
  If Action Subsystem6/1(Out1) -> Merge/7
  Switch Case/1 -> If Action Subsystem/Action
  Switch Case/7 -> If Action Subsystem6/Action
  Switch Case/8 -> If Action Subsystem7/Action
  Switch Case/10 -> If Action Subsystem10/Action
  Switch Case/3 -> If Action Subsystem2/Action
  Switch Case/4 -> If Action Subsystem3/Action
  If Action Subsystem4/1(Out1) -> Merge/5
  Switch Case/6 -> If Action Subsystem5/Action
  If Action Subsystem7/1(Out1) -> Merge/8
  Switch Case/9 -> If Action Subsystem8/Action
  Switch Case/5 -> If Action Subsystem4/Action
  Switch Case/2 -> If Action Subsystem1/Action
  If Action Subsystem3/1(Out1) -> Merge/4

== system top_level_algo/7seg Driver/HR Encoding/7seg encoder/If Action Subsystem ==
  Action Port : ActionPort  ActionPortLabel=case [ 0 ]:
  Constant : Constant  Value=0x3F
  Out1 : Outport
  wires:
  Constant/1 -> Out1/1

== system top_level_algo/7seg Driver/HR Encoding/7seg encoder/If Action Subsystem1 ==
  Action Port : ActionPort  ActionPortLabel=case [ 1 ]:
  Constant : Constant  Value=0x06
  Out1 : Outport
  wires:
  Constant/1 -> Out1/1

== system top_level_algo/7seg Driver/HR Encoding/7seg encoder/If Action Subsystem10 ==
  Action Port : ActionPort  ActionPortLabel=case [ 9 ]:
  Constant : Constant  Value=0x6F
  Out1 : Outport
  wires:
  Constant/1 -> Out1/1

== system top_level_algo/7seg Driver/HR Encoding/7seg encoder/If Action Subsystem2 ==
  Action Port : ActionPort  ActionPortLabel=case [ 2 ]:
  Constant : Constant  Value=0x5B
  Out1 : Outport
  wires:
  Constant/1 -> Out1/1

== system top_level_algo/7seg Driver/HR Encoding/7seg encoder/If Action Subsystem3 ==
  Action Port : ActionPort  ActionPortLabel=case [ 3 ]:
  Constant : Constant  Value=0x4F
  Out1 : Outport
  wires:
  Constant/1 -> Out1/1

== system top_level_algo/7seg Driver/HR Encoding/7seg encoder/If Action Subsystem4 ==
  Action Port : ActionPort  ActionPortLabel=case [ 4 ]:
  Constant : Constant  Value=0x66
  Out1 : Outport
  wires:
  Constant/1 -> Out1/1

== system top_level_algo/7seg Driver/HR Encoding/7seg encoder/If Action Subsystem5 ==
  Action Port : ActionPort  ActionPortLabel=case [ 5 ]:
  Constant : Constant  Value=0x6D
  Out1 : Outport
  wires:
  Constant/1 -> Out1/1

== system top_level_algo/7seg Driver/HR Encoding/7seg encoder/If Action Subsystem6 ==
  Action Port : ActionPort  ActionPortLabel=case [ 6 ]:
  Constant : Constant  Value=0x7D
  Out1 : Outport
  wires:
  Constant/1 -> Out1/1

== system top_level_algo/7seg Driver/HR Encoding/7seg encoder/If Action Subsystem7 ==
  Action Port : ActionPort  ActionPortLabel=case [ 7 ]:
  Constant : Constant  Value=0x07
  Out1 : Outport
  wires:
  Constant/1 -> Out1/1

== system top_level_algo/7seg Driver/HR Encoding/7seg encoder/If Action Subsystem8 ==
  Action Port : ActionPort  ActionPortLabel=case [ 8 ]:
  Constant : Constant  Value=0x7F
  Out1 : Outport
  wires:
  Constant/1 -> Out1/1

== system top_level_algo/7seg Driver/HR Encoding/7seg encoder1/If Action Subsystem ==
  Action Port : ActionPort  ActionPortLabel=case [ 0 ]:
  Constant : Constant  Value=0x3F
  Out1 : Outport
  wires:
  Constant/1 -> Out1/1

== system top_level_algo/7seg Driver/HR Encoding/7seg encoder1/If Action Subsystem1 ==
  Action Port : ActionPort  ActionPortLabel=case [ 1 ]:
  Constant : Constant  Value=0x06
  Out1 : Outport
  wires:
  Constant/1 -> Out1/1

== system top_level_algo/7seg Driver/HR Encoding/7seg encoder1/If Action Subsystem10 ==
  Action Port : ActionPort  ActionPortLabel=case [ 9 ]:
  Constant : Constant  Value=0x6F
  Out1 : Outport
  wires:
  Constant/1 -> Out1/1

== system top_level_algo/7seg Driver/HR Encoding/7seg encoder1/If Action Subsystem2 ==
  Action Port : ActionPort  ActionPortLabel=case [ 2 ]:
  Constant : Constant  Value=0x5B
  Out1 : Outport
  wires:
  Constant/1 -> Out1/1

== system top_level_algo/7seg Driver/HR Encoding/7seg encoder1/If Action Subsystem3 ==
  Action Port : ActionPort  ActionPortLabel=case [ 3 ]:
  Constant : Constant  Value=0x4F
  Out1 : Outport
  wires:
  Constant/1 -> Out1/1

== system top_level_algo/7seg Driver/HR Encoding/7seg encoder1/If Action Subsystem4 ==
  Action Port : ActionPort  ActionPortLabel=case [ 4 ]:
  Constant : Constant  Value=0x66
  Out1 : Outport
  wires:
  Constant/1 -> Out1/1

== system top_level_algo/7seg Driver/HR Encoding/7seg encoder1/If Action Subsystem5 ==
  Action Port : ActionPort  ActionPortLabel=case [ 5 ]:
  Constant : Constant  Value=0x6D
  Out1 : Outport
  wires:
  Constant/1 -> Out1/1

== system top_level_algo/7seg Driver/HR Encoding/7seg encoder1/If Action Subsystem6 ==
  Action Port : ActionPort  ActionPortLabel=case [ 6 ]:
  Constant : Constant  Value=0x7D
  Out1 : Outport
  wires:
  Constant/1 -> Out1/1

== system top_level_algo/7seg Driver/HR Encoding/7seg encoder1/If Action Subsystem7 ==
  Action Port : ActionPort  ActionPortLabel=case [ 7 ]:
  Constant : Constant  Value=0x07
  Out1 : Outport
  wires:
  Constant/1 -> Out1/1

== system top_level_algo/7seg Driver/HR Encoding/7seg encoder1/If Action Subsystem8 ==
  Action Port : ActionPort  ActionPortLabel=case [ 8 ]:
  Constant : Constant  Value=0x7F
  Out1 : Outport
  wires:
  Constant/1 -> Out1/1

== system top_level_algo/7seg Driver/HR Encoding/7seg encoder2/If Action Subsystem ==
  Action Port : ActionPort  ActionPortLabel=case [ 0 ]:
  Constant : Constant  Value=0x3F
  Out1 : Outport
  wires:
  Constant/1 -> Out1/1

== system top_level_algo/7seg Driver/HR Encoding/7seg encoder2/If Action Subsystem1 ==
  Action Port : ActionPort  ActionPortLabel=case [ 1 ]:
  Constant : Constant  Value=0x06
  Out1 : Outport
  wires:
  Constant/1 -> Out1/1

== system top_level_algo/7seg Driver/HR Encoding/7seg encoder2/If Action Subsystem10 ==
  Action Port : ActionPort  ActionPortLabel=case [ 9 ]:
  Constant : Constant  Value=0x6F
  Out1 : Outport
  wires:
  Constant/1 -> Out1/1

== system top_level_algo/7seg Driver/HR Encoding/7seg encoder2/If Action Subsystem2 ==
  Action Port : ActionPort  ActionPortLabel=case [ 2 ]:
  Constant : Constant  Value=0x5B
  Out1 : Outport
  wires:
  Constant/1 -> Out1/1

== system top_level_algo/7seg Driver/HR Encoding/7seg encoder2/If Action Subsystem3 ==
  Action Port : ActionPort  ActionPortLabel=case [ 3 ]:
  Constant : Constant  Value=0x4F
  Out1 : Outport
  wires:
  Constant/1 -> Out1/1

== system top_level_algo/7seg Driver/HR Encoding/7seg encoder2/If Action Subsystem4 ==
  Action Port : ActionPort  ActionPortLabel=case [ 4 ]:
  Constant : Constant  Value=0x66
  Out1 : Outport
  wires:
  Constant/1 -> Out1/1

== system top_level_algo/7seg Driver/HR Encoding/7seg encoder2/If Action Subsystem5 ==
  Action Port : ActionPort  ActionPortLabel=case [ 5 ]:
  Constant : Constant  Value=0x6D
  Out1 : Outport
  wires:
  Constant/1 -> Out1/1

== system top_level_algo/7seg Driver/HR Encoding/7seg encoder2/If Action Subsystem6 ==
  Action Port : ActionPort  ActionPortLabel=case [ 6 ]:
  Constant : Constant  Value=0x7D
  Out1 : Outport
  wires:
  Constant/1 -> Out1/1

== system top_level_algo/7seg Driver/HR Encoding/7seg encoder2/If Action Subsystem7 ==
  Action Port : ActionPort  ActionPortLabel=case [ 7 ]:
  Constant : Constant  Value=0x07
  Out1 : Outport
  wires:
  Constant/1 -> Out1/1

== system top_level_algo/7seg Driver/HR Encoding/7seg encoder2/If Action Subsystem8 ==
  Action Port : ActionPort  ActionPortLabel=case [ 8 ]:
  Constant : Constant  Value=0x7F
  Out1 : Outport
  wires:
  Constant/1 -> Out1/1

== system top_level_algo/7seg Driver/HR Encoding/old encoder3/If Action Subsystem ==
  Action Port : ActionPort
  Constant : Constant  Value=0x3F
  Out1 : Outport
  wires:
  Constant/1 -> Out1/1

== system top_level_algo/7seg Driver/HR Encoding/old encoder3/If Action Subsystem1 ==
  Action Port : ActionPort
  Constant : Constant  Value=0x06
  Out1 : Outport
  wires:
  Constant/1 -> Out1/1

== system top_level_algo/7seg Driver/HR Encoding/old encoder3/If Action Subsystem10 ==
  Action Port : ActionPort
  Constant : Constant  Value=0x6F
  Out1 : Outport
  wires:
  Constant/1 -> Out1/1

== system top_level_algo/7seg Driver/HR Encoding/old encoder3/If Action Subsystem2 ==
  Action Port : ActionPort
  Constant : Constant  Value=0x5B
  Out1 : Outport
  wires:
  Constant/1 -> Out1/1

== system top_level_algo/7seg Driver/HR Encoding/old encoder3/If Action Subsystem3 ==
  Action Port : ActionPort
  Constant : Constant  Value=0x4F
  Out1 : Outport
  wires:
  Constant/1 -> Out1/1

== system top_level_algo/7seg Driver/HR Encoding/old encoder3/If Action Subsystem4 ==
  Action Port : ActionPort
  Constant : Constant  Value=0x66
  Out1 : Outport
  wires:
  Constant/1 -> Out1/1

== system top_level_algo/7seg Driver/HR Encoding/old encoder3/If Action Subsystem5 ==
  Action Port : ActionPort
  Constant : Constant  Value=0x6D
  Out1 : Outport
  wires:
  Constant/1 -> Out1/1

== system top_level_algo/7seg Driver/HR Encoding/old encoder3/If Action Subsystem6 ==
  Action Port : ActionPort
  Constant : Constant  Value=0x7D
  Out1 : Outport
  wires:
  Constant/1 -> Out1/1

== system top_level_algo/7seg Driver/HR Encoding/old encoder3/If Action Subsystem7 ==
  Action Port : ActionPort
  Constant : Constant  Value=0x07
  Out1 : Outport
  wires:
  Constant/1 -> Out1/1

== system top_level_algo/7seg Driver/HR Encoding/old encoder3/If Action Subsystem8 ==
  Action Port : ActionPort
  Constant : Constant  Value=0x7F
  Out1 : Outport
  wires:
  Constant/1 -> Out1/1

== system top_level_algo/7seg Driver2/HR Encoding/7seg encoder/If Action Subsystem ==
  Action Port : ActionPort  ActionPortLabel=case [ 0 ]:
  Constant : Constant  Value=0x3F
  Out1 : Outport
  wires:
  Constant/1 -> Out1/1

== system top_level_algo/7seg Driver2/HR Encoding/7seg encoder/If Action Subsystem1 ==
  Action Port : ActionPort  ActionPortLabel=case [ 1 ]:
  Constant : Constant  Value=0x06
  Out1 : Outport
  wires:
  Constant/1 -> Out1/1

== system top_level_algo/7seg Driver2/HR Encoding/7seg encoder/If Action Subsystem10 ==
  Action Port : ActionPort  ActionPortLabel=case [ 9 ]:
  Constant : Constant  Value=0x6F
  Out1 : Outport
  wires:
  Constant/1 -> Out1/1

== system top_level_algo/7seg Driver2/HR Encoding/7seg encoder/If Action Subsystem2 ==
  Action Port : ActionPort  ActionPortLabel=case [ 2 ]:
  Constant : Constant  Value=0x5B
  Out1 : Outport
  wires:
  Constant/1 -> Out1/1

== system top_level_algo/7seg Driver2/HR Encoding/7seg encoder/If Action Subsystem3 ==
  Action Port : ActionPort  ActionPortLabel=case [ 3 ]:
  Constant : Constant  Value=0x4F
  Out1 : Outport
  wires:
  Constant/1 -> Out1/1

== system top_level_algo/7seg Driver2/HR Encoding/7seg encoder/If Action Subsystem4 ==
  Action Port : ActionPort  ActionPortLabel=case [ 4 ]:
  Constant : Constant  Value=0x66
  Out1 : Outport
  wires:
  Constant/1 -> Out1/1

== system top_level_algo/7seg Driver2/HR Encoding/7seg encoder/If Action Subsystem5 ==
  Action Port : ActionPort  ActionPortLabel=case [ 5 ]:
  Constant : Constant  Value=0x6D
  Out1 : Outport
  wires:
  Constant/1 -> Out1/1

== system top_level_algo/7seg Driver2/HR Encoding/7seg encoder/If Action Subsystem6 ==
  Action Port : ActionPort  ActionPortLabel=case [ 6 ]:
  Constant : Constant  Value=0x7D
  Out1 : Outport
  wires:
  Constant/1 -> Out1/1

== system top_level_algo/7seg Driver2/HR Encoding/7seg encoder/If Action Subsystem7 ==
  Action Port : ActionPort  ActionPortLabel=case [ 7 ]:
  Constant : Constant  Value=0x07
  Out1 : Outport
  wires:
  Constant/1 -> Out1/1

== system top_level_algo/7seg Driver2/HR Encoding/7seg encoder/If Action Subsystem8 ==
  Action Port : ActionPort  ActionPortLabel=case [ 8 ]:
  Constant : Constant  Value=0x7F
  Out1 : Outport
  wires:
  Constant/1 -> Out1/1

== system top_level_algo/7seg Driver2/HR Encoding/7seg encoder1/If Action Subsystem ==
  Action Port : ActionPort  ActionPortLabel=case [ 0 ]:
  Constant : Constant  Value=0x3F
  Out1 : Outport
  wires:
  Constant/1 -> Out1/1

== system top_level_algo/7seg Driver2/HR Encoding/7seg encoder1/If Action Subsystem1 ==
  Action Port : ActionPort  ActionPortLabel=case [ 1 ]:
  Constant : Constant  Value=0x06
  Out1 : Outport
  wires:
  Constant/1 -> Out1/1

== system top_level_algo/7seg Driver2/HR Encoding/7seg encoder1/If Action Subsystem10 ==
  Action Port : ActionPort  ActionPortLabel=case [ 9 ]:
  Constant : Constant  Value=0x6F
  Out1 : Outport
  wires:
  Constant/1 -> Out1/1

== system top_level_algo/7seg Driver2/HR Encoding/7seg encoder1/If Action Subsystem2 ==
  Action Port : ActionPort  ActionPortLabel=case [ 2 ]:
  Constant : Constant  Value=0x5B
  Out1 : Outport
  wires:
  Constant/1 -> Out1/1

== system top_level_algo/7seg Driver2/HR Encoding/7seg encoder1/If Action Subsystem3 ==
  Action Port : ActionPort  ActionPortLabel=case [ 3 ]:
  Constant : Constant  Value=0x4F
  Out1 : Outport
  wires:
  Constant/1 -> Out1/1

== system top_level_algo/7seg Driver2/HR Encoding/7seg encoder1/If Action Subsystem4 ==
  Action Port : ActionPort  ActionPortLabel=case [ 4 ]:
  Constant : Constant  Value=0x66
  Out1 : Outport
  wires:
  Constant/1 -> Out1/1

== system top_level_algo/7seg Driver2/HR Encoding/7seg encoder1/If Action Subsystem5 ==
  Action Port : ActionPort  ActionPortLabel=case [ 5 ]:
  Constant : Constant  Value=0x6D
  Out1 : Outport
  wires:
  Constant/1 -> Out1/1

== system top_level_algo/7seg Driver2/HR Encoding/7seg encoder1/If Action Subsystem6 ==
  Action Port : ActionPort  ActionPortLabel=case [ 6 ]:
  Constant : Constant  Value=0x7D
  Out1 : Outport
  wires:
  Constant/1 -> Out1/1

== system top_level_algo/7seg Driver2/HR Encoding/7seg encoder1/If Action Subsystem7 ==
  Action Port : ActionPort  ActionPortLabel=case [ 7 ]:
  Constant : Constant  Value=0x07
  Out1 : Outport
  wires:
  Constant/1 -> Out1/1

== system top_level_algo/7seg Driver2/HR Encoding/7seg encoder1/If Action Subsystem8 ==
  Action Port : ActionPort  ActionPortLabel=case [ 8 ]:
  Constant : Constant  Value=0x7F
  Out1 : Outport
  wires:
  Constant/1 -> Out1/1

== system top_level_algo/7seg Driver2/HR Encoding/7seg encoder2/If Action Subsystem ==
  Action Port : ActionPort  ActionPortLabel=case [ 0 ]:
  Constant : Constant  Value=0x3F
  Out1 : Outport
  wires:
  Constant/1 -> Out1/1

== system top_level_algo/7seg Driver2/HR Encoding/7seg encoder2/If Action Subsystem1 ==
  Action Port : ActionPort  ActionPortLabel=case [ 1 ]:
  Constant : Constant  Value=0x06
  Out1 : Outport
  wires:
  Constant/1 -> Out1/1
